simulink model "uav_plant_io"  (R2026a)
settings: Solver=ode4  StopTime=50  FixedStep=0.004
undefined symbols (not defined in the file or in its folder): controlParams, eQ, eT, GravityAcc, kQ, kT, Mass, minPWM, rotorsSpeedDown, rotorsSpeedUp, SampleTime, uavParam
libraries: slpidlib x24, simulink x11, robotcorelib x4, matrix_library x4, aerolibasang x4, aerolibobsolete x1, uavutilslib x1
(part 1 of 3)
settings Model: Creator=abutf  LastModifiedBy=Aaron

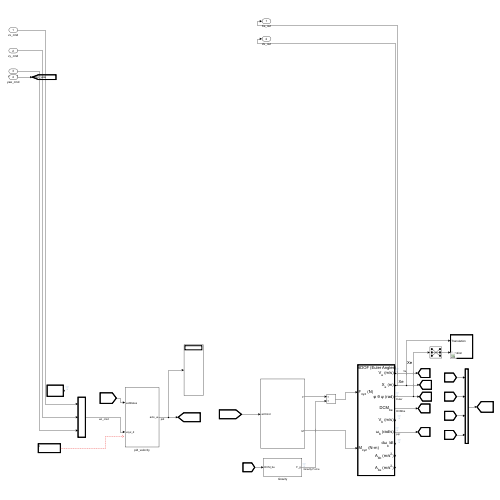
[thumbnail: Simulink's stored preview of the top-level diagram]
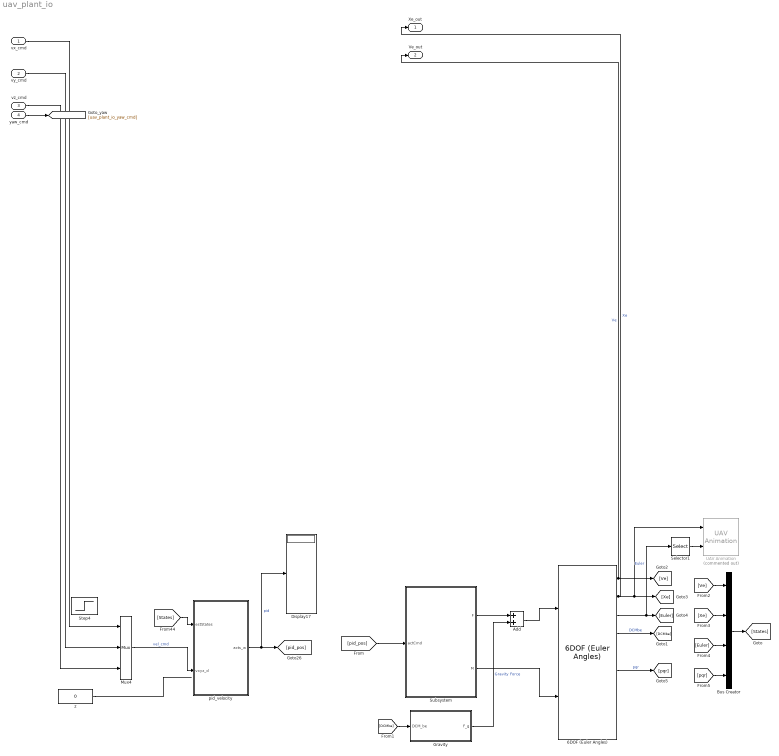
== system uav_plant_io ==
  vx_cmd : Inport
  vy_cmd : Inport  Port=2
  vz_cmd : Inport  Port=3
  yaw_cmd : Inport  Port=4
  6DOF (Euler Angles) : aerolibobsolete/6DOF (Euler Angles)  units=Metric (MKS)  mtype=Fixed  rep=Euler Angles  xme_0=[0, 0, 0]  Vm_0=[0 0 0]  eul_0=[0 0 0]  pm_0=[0 0 0]  mass_0=Mass  mass_e=0.5  mass_f=2.0  inertia=momentInertia  inertia_e=eye(3)  inertia_f=2*eye(3)  k_quat=1.0  vre_flag=on  abi_flag=on  aMode=0  xme_statename=''  Vm_statename=''  eul_statename=''  quat_statename=''  pm_statename=''  mass_statename=''
  Add : Sum
  Bus Creator : BusCreator  Inputs=4
  Display17 : Display
  Gravity : Subsystem
  Mux4 : Mux  Inputs=3
  Selector1 : Selector  InputPortWidth=3  IndexOptions=Index vector (dialog)  Indices=[3 2 1]  OutputSizes=1
  Step4 : Step  Time=5  SampleTime=0
  Subsystem : Subsystem
  UAV Animation : uavutilslib/UAV Animation  Commented=on  NumUAV=1  DynamicUAVConfig=off  UAVType=Multirotor  UAVSize=5  UAVColor=[1 0 0]  UAVTrajectoryAlpha=1  AlwaysShowAnimation=on  AxisLimits=[-Inf Inf;-Inf Inf;-Inf Inf]  TrajectoryBufferSize=100000  InertialZDirection=Down  RotationFormat=Euler ZYX  DrawMarkers=off  SampleTime=-1
  pid_velocity : Subsystem
  z : Constant  Value=0
  Xe_out : Outport
  Ve_out : Outport  Port=2
  wires:
  Mux4/1 -> pid_velocity/2(vxyz_d)  "vel_cmd"
  z/1 -> ?
  [States] -> pid_velocity/1(estStates)
  pid_velocity/1(acts_w) -> [pid_pos], Display17/1  "pid"
  [pid_pos] -> Subsystem/1(actCmd)
  Add/1 -> 6DOF (Euler Angles)/1
  Subsystem/1(F) -> Add/1
  Gravity/1(F_g) -> Add/2  "Gravity Force"
  Subsystem/2(M) -> 6DOF (Euler Angles)/2
  Bus Creator/1 -> [States]
  6DOF (Euler Angles)/4 -> [DCMbe]  "DCMbe"
  [DCMbe] -> Gravity/1(DCM_be)
  6DOF (Euler Angles)/1 -> [Ve], Ve_out/1  "Ve"
  [Ve] -> Bus Creator/1
  [Xe] -> Bus Creator/2
  6DOF (Euler Angles)/3 -> Selector1/1, [Euler]  "Euler"
  [Euler] -> Bus Creator/3
  6DOF (Euler Angles)/6 -> [pqr]  "pqr"
  [pqr] -> Bus Creator/4
  6DOF (Euler Angles)/2 -> UAV Animation/1, [Xe], Xe_out/1  "Xe"
  Selector1/1 -> UAV Animation/2
  vx_cmd/1 -> Mux4/1
  vy_cmd/1 -> Mux4/2
  vz_cmd/1 -> Mux4/3
  yaw_cmd/1 -> [uav_plant_io_yaw_cmd]

== system uav_plant_io/Gravity ==
  DCM_be : Inport
  Constant : Constant  Value=[0 0 GravityAcc]'
  Display4 : Display
  Gain : Gain  Gain=Mass
  Matrix Multiply : Product  Multiplication=Matrix(*)
  F_g : Outport
  wires:
  Matrix Multiply/1 -> Gain/1
  Constant/1 -> Matrix Multiply/2
  DCM_be/1 -> Matrix Multiply/1
  Gain/1 -> Display4/1, F_g/1

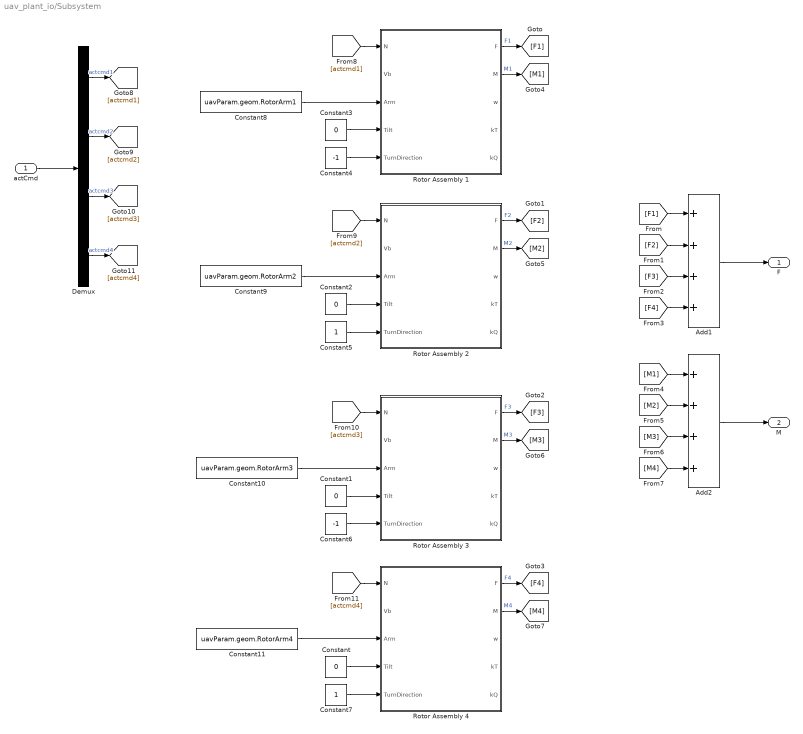
== system uav_plant_io/Subsystem ==
  actCmd : Inport
  Add1 : Sum  Inputs=++++
  Add2 : Sum  Inputs=++++
  Constant{,1..3} (4 alike) : Constant  Value=0
  Constant10 : Constant  Value=uavParam.geom.RotorArm3
  Constant11 : Constant  Value=uavParam.geom.RotorArm4
  Constant4 : Constant  Value=-1
  Constant5 : Constant
  Constant6 : Constant  Value=-1
  Constant7 : Constant
  Constant8 : Constant  Value=uavParam.geom.RotorArm1
  Constant9 : Constant  Value=uavParam.geom.RotorArm2
  Demux : Demux
  Rotor Assembly 1 : Subsystem
  Rotor Assembly 2 : Subsystem
  Rotor Assembly 3 : Subsystem
  Rotor Assembly 4 : Subsystem
  F : Outport
  M : Outport  Port=2
  wires:
  Constant10/1 -> Rotor Assembly 3/3(Arm)
  Add1/1 -> F/1
  ? -> Rotor Assembly 3/2(Vb)
  Constant6/1 -> Rotor Assembly 3/5(TurnDirection)
  Constant1/1 -> Rotor Assembly 3/4(Tilt)
  Add2/1 -> M/1
  Constant/1 -> Rotor Assembly 4/4(Tilt)
  Constant2/1 -> Rotor Assembly 2/4(Tilt)
  Constant3/1 -> Rotor Assembly 1/4(Tilt)
  Constant4/1 -> Rotor Assembly 1/5(TurnDirection)
  Constant5/1 -> Rotor Assembly 2/5(TurnDirection)
  Constant7/1 -> Rotor Assembly 4/5(TurnDirection)
  Constant8/1 -> Rotor Assembly 1/3(Arm)
  Constant9/1 -> Rotor Assembly 2/3(Arm)
  Constant11/1 -> Rotor Assembly 4/3(Arm)
  Rotor Assembly 1/1(F) -> [F1]  "F1"
  [F1] -> Add1/1
  Rotor Assembly 2/1(F) -> [F2]  "F2"
  [F2] -> Add1/2
  Rotor Assembly 3/1(F) -> [F3]  "F3"
  [F3] -> Add1/3
  Rotor Assembly 4/1(F) -> [F4]  "F4"
  [F4] -> Add1/4
  Rotor Assembly 1/2(M) -> [M1]  "M1"
  [M1] -> Add2/1
  Rotor Assembly 2/2(M) -> [M2]  "M2"
  [M2] -> Add2/2
  Rotor Assembly 3/2(M) -> [M3]  "M3"
  [M3] -> Add2/3
  Rotor Assembly 4/2(M) -> [M4]  "M4"
  [M4] -> Add2/4
  actCmd/1 -> Demux/1
  Demux/1 -> [actcmd1]  "actcmd1"
  [actcmd1] -> Rotor Assembly 1/1(N)
  Demux/2 -> [actcmd2]  "actcmd2"
  [actcmd2] -> Rotor Assembly 2/1(N)
  Demux/3 -> [actcmd3]  "actcmd3"
  [actcmd3] -> Rotor Assembly 3/1(N)
  Demux/4 -> [actcmd4]  "actcmd4"
  [actcmd4] -> Rotor Assembly 4/1(N)

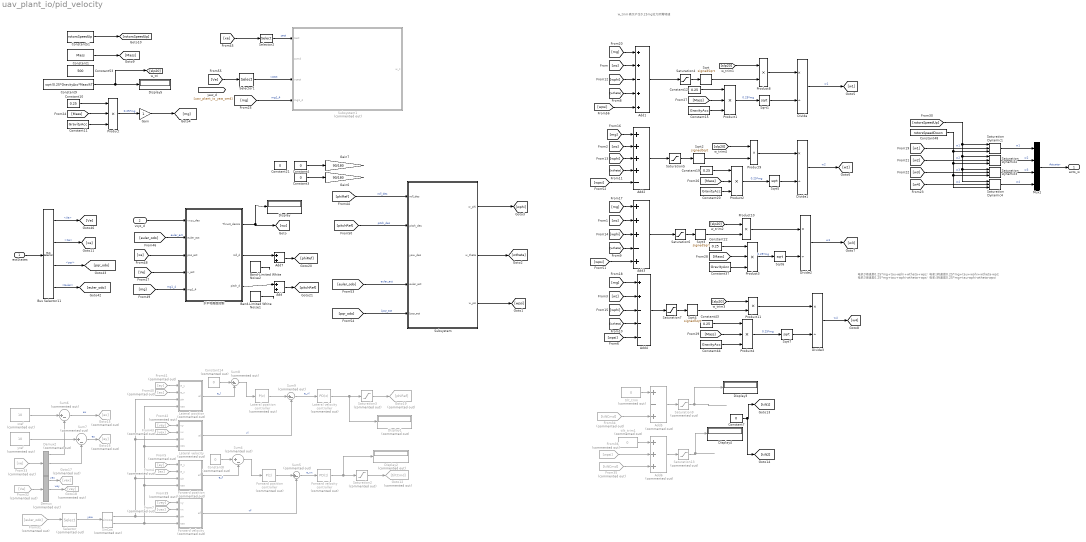
== system uav_plant_io/pid_velocity ==
  note: 电机1转速是0.25*mg+tau-wphi+wtheta+wpsi，
      | 电机2转速是0.25*mg+tau+wphi+wtheta-wpsi，
      | 电机3转速是0.25*mg+tau+wphi-wtheta+wpsi，
      | 电机4转速是0.25*mg+tau-wphi-wtheta-wpsi
  note: w_trim 表示产生0.25mg拉力所需转速
  estStates : Inport
  vxyz_d : Inport  Port=2
  Add : Sum
  Add1 : Sum  Inputs=++-++
  Add2 : Sum  Inputs=++++-
  Add3 : Sum  Inputs=+++-+
  Add4 : Sum  Inputs=++---
  Add5 : Sum  Commented=on  Inputs=+-+
  Add6 : Sum  Commented=on  Inputs=+++
  Add7 : Sum
  Band-Limited White Noise1 : simulink/Sources/Band-Limited White Noise  Cov=[0.000001]  Ts=SampleTime  seed=[23341]
  Band-Limited White Noise2 : simulink/Sources/Band-Limited White Noise  Cov=[0.000001]  Ts=SampleTime  seed=[2341]
  Bus Selector11 : BusSelector  OutputSignals=Ve,Xe,pqr,Euler
  Constant1 : Constant  Value=Mass  OutDataTypeStr=double
  Constant{10,12,19,22,43} (5 alike) : Constant  Value=0.25  OutDataTypeStr=double
  Constant{11,15,20,37,44} (5 alike) : Constant  Value=GravityAcc  OutDataTypeStr=double
  Constant14 : Constant  Commented=on  Value=0
  Constant{3..4,7,21} (4 alike) : Constant  Value=0  OutDataTypeStr=double
  Constant48 : Constant  Value=rotorsSpeedDown  OutDataTypeStr=double
  Constant51 : Constant  Value=rotorsSpeedUp  OutDataTypeStr=double
  Constant53 : Constant  Value=500
  Constant8 : Constant  Commented=on  Value=0
  Constant9 : Constant  Value=sqrt(0.25*GravityAcc*Mass/kT)
  Demux : Demux  Commented=on  Outputs=3
  Demux2 : Demux  Commented=on  Outputs=3
  Display{,3..5} (4 alike) : Display
  Display1 : Display  Commented=on
  Display2 : Display  Commented=on
  Divide{,1..3} (4 alike) : Product  Inputs=*/
  Forward position : Subsystem  Commented=on
  Forward position controller : slpidlib/PID Controller  Commented=on  Controller=P  Form=Parallel  TimeDomain=Discrete-time  UseExternalTs=off  SampleTime=-1  IntegratorMethod=Forward Euler  FilterMethod=Forward Euler  ControllerParametersSource=internal  P=1  I=controlParams.I_X  UseKiTs=off  D=0.741088334151374  UseExternalDerivativeSource=off  N=1.14081860742283  UseFilter=on  TunerSelectOption=Transfer Function Based (PID Tuner App)  InitialConditionSource=internal  InitialConditionForIntegrator=0  InitialConditionForFilter=0  DifferentiatorICPrevScaledInput=0  ExternalReset=none  TrackingMode=off  Kt=1  LimitOutput=off  SatLimitsSource=internal  UpperSaturationLimit=inf  LowerSaturationLimit=-inf  LinearizeAsGain=on  AntiWindupMode=none  Kb=1  LimitIntegrator=off  UpperIntegratorSaturationLimit=inf  LowerIntegratorSaturationLimit=-inf  POutMin=[]  POutMax=[]  IOutMin=[]  IOutMax=[]  DOutMin=[]  DOutMax=[]  NOutMin=[]  NOutMax=[]  SumOutMin=[]  SumOutMax=[]  SaturationOutMin=[]  SaturationOutMax=[]  PParamMin=[]  PParamMax=[]  IParamMin=[]  IParamMax=[]  DParamMin=[]  DParamMax=[]  NParamMin=[]  NParamMax=[]  KbParamMin=[]  KbParamMax=[]  KtParamMin=[]  KtParamMax=[]  KbOutMin=[]  KbOutMax=[]  KtOutMin=[]  KtOutMax=[]  IntegratorOutMin=[]  IntegratorOutMax=[]  FilterOutMin=[]  FilterOutMax=[]  SumI1OutMin=[]  SumI1OutMax=[]  SumI2OutMin=[]  SumI2OutMax=[]  SumI3OutMin=[]  SumI3OutMax=[]  SumI4OutMin=[]  SumI4OutMax=[]  SumDOutMin=[]  SumDOutMax=[]  DifferentiatorOutMin=[]  DifferentiatorOutMax=[]  FilterDiffOutCoefMin=[]  FilterDiffOutCoefMax=[]  ReciprocalOutMin=[]  ReciprocalOutMax=[]  SumDenOutMin=[]  SumDenOutMax=[]  SumNumOutMin=[]  SumNumOutMax=[]  DivideOutMin=[]  DivideOutMax=[]  UdiffTsProdOutMin=[]  UdiffTsProdOutMax=[]  NTsProdOutMin=[]  NTsProdOutMax=[]  UintegralTsProdOutMin=[]  UintegralTsProdOutMax=[]  UngainTsProdOutMin=[]  UngainTsProdOutMax=[]  ClampingZeroOutDataTypeStr=Inherit: Inherit via back propagation  ClampingZeroOutMin=[]  ClampingZeroOutMax=[]  FilterDenConstantOutDataTypeStr=Inherit: Inherit via back propagation  FilterDenConstantOutMin=[]  FilterDenConstantOutMax=[]  PCopyOutDataTypeStr=Inherit: Inherit via back propagation  PCopyOutMin=[]  PCopyOutMax=[]  NCopyOutDataTypeStr=Inherit: Inherit via back propagation  NCopyOutMin=[]  NCopyOutMax=[]  IntegratorContinuousStateAttributes=''  IntegratorStateMustResolveToSignalObject=off  IntegratorRTWStateStorageClass=Auto  FilterContinuousStateAttributes=''  FilterStateMustResolveToSignalObject=off  FilterRTWStateStorageClass=Auto  ParallelPVariant=InternalParameters  IdealPVariant=Disabled  IVariant=Disabled  DVariant=Disabled  IntegratorVariant=Disabled  SatVariant=Disabled  AWVariant=Disabled  PCopyVariant=Disabled  TRVariant=Disabled  FdbkBlocksVariant=Forward  IdealPFdbkVariant=Disabled  SatFdbkVariant=Disabled  DerivativeFilterVariant=Disabled  NVariant=Disabled  NCopyVariant=Disabled_SignalSpec  FilterICVariant=Disabled  IntegratorICVariant=Disabled  ExternalResetVariant=Disabled  TRSumVariant=Passthrough  SumFdbkVariant=Disabled  SumVariant=Passthrough_P  TsampFilterVariant=InternalTs  TsampNgainVariant=Passthrough  TsampIntegralVariant=Disabled_SignalSpec  ExternalSaturationOutDataTypeStr=Inherit: Same as second input  DerivativeSourceVariant=Disabled  PreIntVariant=InternalPreInt
  Forward velocity : Subsystem  Commented=on
  Forward velocity controller : slpidlib/PID Controller  Commented=on  Controller=PD  Form=Parallel  TimeDomain=Discrete-time  UseExternalTs=off  SampleTime=-1  IntegratorMethod=Forward Euler  FilterMethod=Forward Euler  ControllerParametersSource=internal  P=10  I=0  UseKiTs=off  D=0.1  UseExternalDerivativeSource=off  N=20  UseFilter=on  TunerSelectOption=Transfer Function Based (PID Tuner App)  InitialConditionSource=internal  InitialConditionForIntegrator=0  InitialConditionForFilter=0  DifferentiatorICPrevScaledInput=0  ExternalReset=none  TrackingMode=off  Kt=1  LimitOutput=off  SatLimitsSource=internal  UpperSaturationLimit=inf  LowerSaturationLimit=-inf  LinearizeAsGain=on  AntiWindupMode=none  Kb=1  LimitIntegrator=off  UpperIntegratorSaturationLimit=inf  LowerIntegratorSaturationLimit=-inf  POutMin=[]  POutMax=[]  IOutMin=[]  IOutMax=[]  DOutMin=[]  DOutMax=[]  NOutMin=[]  NOutMax=[]  SumOutMin=[]  SumOutMax=[]  SaturationOutMin=[]  SaturationOutMax=[]  PParamMin=[]  PParamMax=[]  IParamMin=[]  IParamMax=[]  DParamMin=[]  DParamMax=[]  NParamMin=[]  NParamMax=[]  KbParamMin=[]  KbParamMax=[]  KtParamMin=[]  KtParamMax=[]  KbOutMin=[]  KbOutMax=[]  KtOutMin=[]  KtOutMax=[]  IntegratorOutMin=[]  IntegratorOutMax=[]  FilterOutMin=[]  FilterOutMax=[]  SumI1OutMin=[]  SumI1OutMax=[]  SumI2OutMin=[]  SumI2OutMax=[]  SumI3OutMin=[]  SumI3OutMax=[]  SumI4OutMin=[]  SumI4OutMax=[]  SumDOutMin=[]  SumDOutMax=[]  DifferentiatorOutMin=[]  DifferentiatorOutMax=[]  FilterDiffOutCoefMin=[]  FilterDiffOutCoefMax=[]  ReciprocalOutMin=[]  ReciprocalOutMax=[]  SumDenOutMin=[]  SumDenOutMax=[]  SumNumOutMin=[]  SumNumOutMax=[]  DivideOutMin=[]  DivideOutMax=[]  UdiffTsProdOutMin=[]  UdiffTsProdOutMax=[]  NTsProdOutMin=[]  NTsProdOutMax=[]  UintegralTsProdOutMin=[]  UintegralTsProdOutMax=[]  UngainTsProdOutMin=[]  UngainTsProdOutMax=[]  ClampingZeroOutDataTypeStr=Inherit: Inherit via back propagation  ClampingZeroOutMin=[]  ClampingZeroOutMax=[]  FilterDenConstantOutDataTypeStr=Inherit: Inherit via back propagation  FilterDenConstantOutMin=[]  FilterDenConstantOutMax=[]  PCopyOutDataTypeStr=Inherit: Inherit via back propagation  PCopyOutMin=[]  PCopyOutMax=[]  NCopyOutDataTypeStr=Inherit: Inherit via back propagation  NCopyOutMin=[]  NCopyOutMax=[]  IntegratorContinuousStateAttributes=''  IntegratorStateMustResolveToSignalObject=off  IntegratorRTWStateStorageClass=Auto  FilterContinuousStateAttributes=''  FilterStateMustResolveToSignalObject=off  FilterRTWStateStorageClass=Auto  ParallelPVariant=InternalParameters  IdealPVariant=Disabled  IVariant=Disabled  DVariant=InternalParameters  IntegratorVariant=Disabled  SatVariant=Disabled  AWVariant=Disabled  PCopyVariant=Disabled  TRVariant=Disabled  FdbkBlocksVariant=Forward  IdealPFdbkVariant=Disabled  SatFdbkVariant=Disabled  DerivativeFilterVariant=ForwardEulerFilter  NVariant=InternalParameters  NCopyVariant=Disabled  FilterICVariant=InternalICsFilter  IntegratorICVariant=Disabled  ExternalResetVariant=Disabled  TRSumVariant=Passthrough  SumFdbkVariant=Disabled  SumVariant=Sum_PD  TsampFilterVariant=InternalTs  TsampNgainVariant=Passthrough  TsampIntegralVariant=Disabled_SignalSpec  ExternalSaturationOutDataTypeStr=Inherit: Same as second input  DerivativeSourceVariant=ErrorSignal  PreIntVariant=InternalPreInt
  From31 : From  Commented=on  GotoTag=euler_odo
  From32 : From  Commented=on  GotoTag=Ve
  From33 : From  Commented=on  GotoTag=xe
  From34 : From  Commented=on  GotoTag=tiltCmd
  From35 : From  Commented=on  GotoTag=tiltCmd
  From36 : From  Commented=on  GotoTag=wpsi
  From39 : From  Commented=on  GotoTag=vey
  From4 : From  Commented=on  GotoTag=ex
  From40 : From  Commented=on  GotoTag=ex
  From41 : From  Commented=on  GotoTag=ey
  From42 : From  Commented=on  GotoTag=vey
  From43 : From  Commented=on  GotoTag=vex
  From5 : From  Commented=on  GotoTag=ey
  From7 : From  Commented=on  GotoTag=vex
  Gain : Gain
  Gain6 : Gain  Gain=90/180
  Gain7 : Gain  Gain=90/180
  Goto12 : Goto  Commented=on  GotoTag=tiltCmd
  Goto15 : Goto  Commented=on  GotoTag=ex
  Goto16 : Goto  Commented=on  GotoTag=ey
  Goto17 : Goto  Commented=on  GotoTag=vex
  Goto18 : Goto  Commented=on  GotoTag=vey
  Goto19 : Goto  Commented=on  GotoTag=phiRef
  Lateral position : Subsystem  Commented=on
  Lateral position controller : slpidlib/PID Controller  Commented=on  Controller=P  Form=Parallel  TimeDomain=Discrete-time  UseExternalTs=off  SampleTime=-1  IntegratorMethod=Forward Euler  FilterMethod=Forward Euler  ControllerParametersSource=internal  P=1  I=controlParams.I_Y  UseKiTs=off  D=0.20966837124708  UseExternalDerivativeSource=off  N=1.18305565097938  UseFilter=on  TunerSelectOption=Transfer Function Based (PID Tuner App)  InitialConditionSource=internal  InitialConditionForIntegrator=0  InitialConditionForFilter=0  DifferentiatorICPrevScaledInput=0  ExternalReset=none  TrackingMode=off  Kt=1  LimitOutput=off  SatLimitsSource=internal  UpperSaturationLimit=0.4  LowerSaturationLimit=-0.4  LinearizeAsGain=on  AntiWindupMode=clamping  Kb=1  LimitIntegrator=off  UpperIntegratorSaturationLimit=inf  LowerIntegratorSaturationLimit=-inf  POutMin=[]  POutMax=[]  IOutMin=[]  IOutMax=[]  DOutMin=[]  DOutMax=[]  NOutMin=[]  NOutMax=[]  SumOutMin=[]  SumOutMax=[]  SaturationOutMin=[]  SaturationOutMax=[]  PParamMin=[]  PParamMax=[]  IParamMin=[]  IParamMax=[]  DParamMin=[]  DParamMax=[]  NParamMin=[]  NParamMax=[]  KbParamMin=[]  KbParamMax=[]  KtParamMin=[]  KtParamMax=[]  KbOutMin=[]  KbOutMax=[]  KtOutMin=[]  KtOutMax=[]  IntegratorOutMin=[]  IntegratorOutMax=[]  FilterOutMin=[]  FilterOutMax=[]  SumI1OutMin=[]  SumI1OutMax=[]  SumI2OutMin=[]  SumI2OutMax=[]  SumI3OutMin=[]  SumI3OutMax=[]  SumI4OutMin=[]  SumI4OutMax=[]  SumDOutMin=[]  SumDOutMax=[]  DifferentiatorOutMin=[]  DifferentiatorOutMax=[]  FilterDiffOutCoefMin=[]  FilterDiffOutCoefMax=[]  ReciprocalOutMin=[]  ReciprocalOutMax=[]  SumDenOutMin=[]  SumDenOutMax=[]  SumNumOutMin=[]  SumNumOutMax=[]  DivideOutMin=[]  DivideOutMax=[]  UdiffTsProdOutMin=[]  UdiffTsProdOutMax=[]  NTsProdOutMin=[]  NTsProdOutMax=[]  UintegralTsProdOutMin=[]  UintegralTsProdOutMax=[]  UngainTsProdOutMin=[]  UngainTsProdOutMax=[]  ClampingZeroOutDataTypeStr=Inherit: Inherit via back propagation  ClampingZeroOutMin=[]  ClampingZeroOutMax=[]  FilterDenConstantOutDataTypeStr=Inherit: Inherit via back propagation  FilterDenConstantOutMin=[]  FilterDenConstantOutMax=[]  PCopyOutDataTypeStr=Inherit: Inherit via back propagation  PCopyOutMin=[]  PCopyOutMax=[]  NCopyOutDataTypeStr=Inherit: Inherit via back propagation  NCopyOutMin=[]  NCopyOutMax=[]  IntegratorContinuousStateAttributes=''  IntegratorStateMustResolveToSignalObject=off  IntegratorRTWStateStorageClass=Auto  FilterContinuousStateAttributes=''  FilterStateMustResolveToSignalObject=off  FilterRTWStateStorageClass=Auto  ParallelPVariant=InternalParameters  IdealPVariant=Disabled  IVariant=Disabled  DVariant=Disabled  IntegratorVariant=Disabled  SatVariant=Disabled  AWVariant=Disabled  PCopyVariant=Disabled  TRVariant=Disabled  FdbkBlocksVariant=Forward  IdealPFdbkVariant=Disabled  SatFdbkVariant=Disabled  DerivativeFilterVariant=Disabled  NVariant=Disabled  NCopyVariant=Disabled_SignalSpec  FilterICVariant=Disabled  IntegratorICVariant=Disabled  ExternalResetVariant=Disabled  TRSumVariant=Passthrough  SumFdbkVariant=Disabled  SumVariant=Passthrough_P  TsampFilterVariant=InternalTs  TsampNgainVariant=Passthrough  TsampIntegralVariant=Disabled_SignalSpec  ExternalSaturationOutDataTypeStr=Inherit: Same as second input  DerivativeSourceVariant=Disabled  PreIntVariant=InternalPreInt
  Lateral velocity : Subsystem  Commented=on
  "Lateral velocity controller " : slpidlib/PID Controller  Commented=on  Controller=PD  Form=Parallel  TimeDomain=Discrete-time  UseExternalTs=off  SampleTime=-1  IntegratorMethod=Forward Euler  FilterMethod=Forward Euler  ControllerParametersSource=internal  P=10  I=0  UseKiTs=off  D=0.1  UseExternalDerivativeSource=off  N=20  UseFilter=on  TunerSelectOption=Transfer Function Based (PID Tuner App)  InitialConditionSource=internal  InitialConditionForIntegrator=0  InitialConditionForFilter=0  DifferentiatorICPrevScaledInput=0  ExternalReset=none  TrackingMode=off  Kt=1  LimitOutput=off  SatLimitsSource=internal  UpperSaturationLimit=inf  LowerSaturationLimit=-inf  LinearizeAsGain=on  AntiWindupMode=none  Kb=1  LimitIntegrator=off  UpperIntegratorSaturationLimit=inf  LowerIntegratorSaturationLimit=-inf  POutMin=[]  POutMax=[]  IOutMin=[]  IOutMax=[]  DOutMin=[]  DOutMax=[]  NOutMin=[]  NOutMax=[]  SumOutMin=[]  SumOutMax=[]  SaturationOutMin=[]  SaturationOutMax=[]  PParamMin=[]  PParamMax=[]  IParamMin=[]  IParamMax=[]  DParamMin=[]  DParamMax=[]  NParamMin=[]  NParamMax=[]  KbParamMin=[]  KbParamMax=[]  KtParamMin=[]  KtParamMax=[]  KbOutMin=[]  KbOutMax=[]  KtOutMin=[]  KtOutMax=[]  IntegratorOutMin=[]  IntegratorOutMax=[]  FilterOutMin=[]  FilterOutMax=[]  SumI1OutMin=[]  SumI1OutMax=[]  SumI2OutMin=[]  SumI2OutMax=[]  SumI3OutMin=[]  SumI3OutMax=[]  SumI4OutMin=[]  SumI4OutMax=[]  SumDOutMin=[]  SumDOutMax=[]  DifferentiatorOutMin=[]  DifferentiatorOutMax=[]  FilterDiffOutCoefMin=[]  FilterDiffOutCoefMax=[]  ReciprocalOutMin=[]  ReciprocalOutMax=[]  SumDenOutMin=[]  SumDenOutMax=[]  SumNumOutMin=[]  SumNumOutMax=[]  DivideOutMin=[]  DivideOutMax=[]  UdiffTsProdOutMin=[]  UdiffTsProdOutMax=[]  NTsProdOutMin=[]  NTsProdOutMax=[]  UintegralTsProdOutMin=[]  UintegralTsProdOutMax=[]  UngainTsProdOutMin=[]  UngainTsProdOutMax=[]  ClampingZeroOutDataTypeStr=Inherit: Inherit via back propagation  ClampingZeroOutMin=[]  ClampingZeroOutMax=[]  FilterDenConstantOutDataTypeStr=Inherit: Inherit via back propagation  FilterDenConstantOutMin=[]  FilterDenConstantOutMax=[]  PCopyOutDataTypeStr=Inherit: Inherit via back propagation  PCopyOutMin=[]  PCopyOutMax=[]  NCopyOutDataTypeStr=Inherit: Inherit via back propagation  NCopyOutMin=[]  NCopyOutMax=[]  IntegratorContinuousStateAttributes=''  IntegratorStateMustResolveToSignalObject=off  IntegratorRTWStateStorageClass=Auto  FilterContinuousStateAttributes=''  FilterStateMustResolveToSignalObject=off  FilterRTWStateStorageClass=Auto  ParallelPVariant=InternalParameters  IdealPVariant=Disabled  IVariant=Disabled  DVariant=InternalParameters  IntegratorVariant=Disabled  SatVariant=Disabled  AWVariant=Disabled  PCopyVariant=Disabled  TRVariant=Disabled  FdbkBlocksVariant=Forward  IdealPFdbkVariant=Disabled  SatFdbkVariant=Disabled  DerivativeFilterVariant=ForwardEulerFilter  NVariant=InternalParameters  NCopyVariant=Disabled  FilterICVariant=InternalICsFilter  IntegratorICVariant=Disabled  ExternalResetVariant=Disabled  TRSumVariant=Passthrough  SumFdbkVariant=Disabled  SumVariant=Sum_PD  TsampFilterVariant=InternalTs  TsampNgainVariant=Passthrough  TsampIntegralVariant=Disabled_SignalSpec  ExternalSaturationOutDataTypeStr=Inherit: Same as second input  DerivativeSourceVariant=ErrorSignal  PreIntVariant=InternalPreInt
  Mux1 : Mux
  Product{,1..4} (5 alike) : Product  Inputs=3
  Product{8..11} (4 alike) : Product
  Saturation Dynamic{1..4} (4 alike) : simulink/Discontinuities/Saturation Dynamic  OutMin=[]  OutMax=[]  OutDataTypeStr=double  OutDataType=fixdt(1, 16)  OutScaling=2^-10  DoSatur=off
  Saturation13 : Saturate  Commented=on  UpperLimit=0.3  LowerLimit=0
  Saturation2 : Saturate  Commented=on  UpperLimit=0.75  LowerLimit=-0.75
  Saturation3 : Saturate  Commented=on  UpperLimit=0.75  LowerLimit=-0.75
  Saturation{4..7} (4 alike) : Saturate  UpperLimit=inf  LowerLimit=0
  Saturation9 : Saturate  Commented=on  UpperLimit=0.3  LowerLimit=0
  Selector : Selector  Commented=on  InputPortWidth=3  IndexOptions=Index vector (dialog)  Indices=[3]  OutputSizes=1
  Selector1 : Selector  InputPortWidth=3  IndexOptions=Index vector (dialog)  Indices=[3]  OutputSizes=1
  Selector2 : Selector  InputPortWidth=3  IndexOptions=Index vector (dialog)  Indices=[3]  OutputSizes=1
  SinCos : Trigonometry  Commented=on  Operator=sincos
  Sqrt{,2..4} (4 alike) : Sqrt  Operator=signedSqrt
  Sqrt{1,5..7} (4 alike) : Sqrt
  Subsystem : Subsystem
  Subsystem1 : Subsystem  Commented=on
  Sum{4..9} (6 alike) : Sum  Commented=on  Inputs=|+-
  tilt_trim : Constant  Commented=on  Value=0
  tilt_trim1 : Constant  Commented=on  Value=0
  xref : Constant  Commented=on  Value=10  OutDataTypeStr=boolean
  yref : Constant  Commented=on  Value=10  OutDataTypeStr=boolean
  水平和高度控制 : Subsystem
  acts_w : Outport
  wires:
  Add7/1 -> [phiRef]
  Band-Limited White Noise2/1 -> ?
  Band-Limited White Noise1/1 -> ?
  Add/1 -> [pitchRef]
  Gain/1 -> [mg]
  Constant7/1 -> [tilt1], [tilt2]
  水平和高度控制/3(pitch_d) -> Add/1
  [mg] -> 水平和高度控制/5(mg1_4)  "mg1_4"
  [mg] -> Subsystem1/4(mg1_4)  "mg1_4"
  Selector1/1 -> Subsystem1/3(vzact)  "vzact"
  ? -> Subsystem1/2(zcmd)  "zcmd"
  Selector2/1 -> Subsystem1/1(zact)  "zact"
  水平和高度控制/1(Thrust_desire) -> [wz], Display/1
  vxyz_d/1 -> 水平和高度控制/1(vxyz_des)
  水平和高度控制/2(roll_d) -> Add7/1
  [xe] -> 水平和高度控制/3(pos_act)
  [Ve] -> 水平和高度控制/4(v_act)
  [euler_odo] -> 水平和高度控制/2(euler_act)  "euler_act"
  Subsystem/3(w_psi) -> [wpsi]
  Subsystem/2(w_theta) -> [wtheta]
  Subsystem/1(w_phi) -> [wphi]
  [pqr_odo] -> Subsystem/5("[pqr_act")  "[pqr_act"
  [euler_odo] -> Subsystem/4(euler_act)  "euler_act"
  [pitchRef] -> Subsystem/2(pitch_des)  "pitch_des"
  [phiRef] -> Subsystem/1(roll_des)  "roll_des"
  Bus Selector11/4 -> [euler_odo]  "<Euler>"
  Bus Selector11/3 -> [pqr_odo]  "<pqr>"
  Bus Selector11/2 -> [xe]  "<Xe>"
  Bus Selector11/1 -> [Ve]  "<Ve>"
  Constant51/1 -> [rotorsSpeedUp]
  Constant9/1 -> [slp20], Display5/1
  Constant1/1 -> [Mass]
  Mux1/1 -> acts_w/1  "Actuator"
  estStates/1 -> Bus Selector11/1
  [w2] -> Saturation Dynamic2/2  "w2"
  [w4] -> Saturation Dynamic4/2  "w4"
  [w3] -> Saturation Dynamic3/2  "w3"
  [w1] -> Saturation Dynamic1/2  "w1"
  [rotorsSpeedUp] -> Saturation Dynamic1/1, Saturation Dynamic2/1, Saturation Dynamic4/1, Saturation Dynamic3/1
  Constant48/1 -> Saturation Dynamic1/3, Saturation Dynamic2/3, Saturation Dynamic4/3, Saturation Dynamic3/3
  [slp20] -> Product11/1
  [slp20] -> Product10/1
  [slp20] -> Product9/1
  [slp20] -> Product8/1
  Sqrt7/1 -> Divide3/2
  Constant44/1 -> Product4/3
  [Mass] -> Product4/2
  Constant43/1 -> Product4/1
  Product4/1 -> Sqrt7/1  "0.25*mg"
  Product11/1 -> Divide3/1
  Product10/1 -> Divide2/1
  Product3/1 -> Sqrt6/1  "0.25*mg"
  Constant22/1 -> Product3/1
  [Mass] -> Product3/2
  Constant37/1 -> Product3/3
  Sqrt6/1 -> Divide2/2
  Sqrt5/1 -> Divide1/2
  Constant20/1 -> Product2/3
  [Mass] -> Product2/2
  Constant19/1 -> Product2/1
  Product2/1 -> Sqrt5/1  "0.25*mg"
  Product9/1 -> Divide1/1
  Product8/1 -> Divide/1
  Product1/1 -> Sqrt1/1  "0.25*mg"
  Constant12/1 -> Product1/1
  [Mass] -> Product1/2
  Constant15/1 -> Product1/3
  Sqrt1/1 -> Divide/2
  Constant11/1 -> Product/3
  [Mass] -> Product/2
  Constant10/1 -> Product/1
  Saturation Dynamic4/1 -> Mux1/4  "w4"
  Saturation Dynamic3/1 -> Mux1/3  "w3"
  Saturation Dynamic2/1 -> Mux1/2  "w2"
  Saturation Dynamic1/1 -> Mux1/1  "w1"
  [Ve] -> Selector1/1
  Divide3/1 -> [w4]  "w4"
  Divide2/1 -> [w3]  "w3"
  Divide1/1 -> [w2]  "w2"
  Divide/1 -> [w1]  "w1"
  [mg] -> Add4/1
  [mg] -> Add2/1
  [mg] -> Add3/1
  [mg] -> Add1/1
  Product/1 -> Gain/1  "0.25*mg"
  [wphi] -> Add4/3
  [wphi] -> Add3/3
  [wphi] -> Add2/3
  [wphi] -> Add1/3
  [wtheta] -> Add2/4
  [wtheta] -> Add4/4
  [wtheta] -> Add3/4
  [wtheta] -> Add1/4
  [wpsi] -> Add2/5
  [wpsi] -> Add4/5
  [wpsi] -> Add1/5
  [wpsi] -> Add3/5
  [wz] -> Add4/2
  [wz] -> Add2/2
  [wz] -> Add3/2
  [wz] -> Add1/2
  Saturation4/1 -> Sqrt/1
  Saturation6/1 -> Sqrt3/1
  Add3/1 -> Saturation6/1
  Add4/1 -> Saturation7/1
  Sqrt/1 -> Product8/2
  Saturation5/1 -> Sqrt2/1
  Add2/1 -> Saturation5/1
  Sqrt4/1 -> Product11/2
  Add1/1 -> Saturation4/1
  Saturation7/1 -> Sqrt4/1
  Sqrt3/1 -> Product10/2
  Sqrt2/1 -> Product9/2
  Constant4/1 -> Gain7/1
  Constant3/1 -> Gain6/1
  Forward position/1(ef) -> Sum4/2  "e_f"
  Sum5/1 -> Forward velocity controller/1  "e_vx"
  Forward velocity controller/1 -> Display2/1, Saturation2/1
  Constant8/1 -> Sum4/1
  Sum4/1 -> Forward position controller/1
  Forward velocity/1(ef) -> Sum5/2  "vf"
  Forward position controller/1 -> Sum5/1
  Selector/1 -> SinCos/1  "yaw"
  SinCos/2 -> Lateral velocity/4(cos), Lateral position/4(cos), Forward position/4(cos), Forward velocity/4(cos)
  SinCos/1 -> Forward velocity/3(sin), Lateral position/3(sin), Lateral velocity/3(sin), Forward position/3(sin)
  From31/1 -> Selector/1
  From32/1 -> Demux/1
  From33/1 -> Demux2/1
  Demux2/1 -> Sum6/2
  Demux2/2 -> Sum7/2
  xref/1 -> Sum6/1
  yref/1 -> Sum7/1
  Saturation2/1 -> Goto12/1
  Saturation9/1 -> Display3/1
  From36/1 -> Add6/2
  tilt_trim1/1 -> Add6/1
  Saturation13/1 -> Display4/1
  From35/1 -> Add6/3
  tilt_trim/1 -> Add5/1
  ? -> Add5/2
  From34/1 -> Add5/3
  Add5/1 -> Saturation9/1
  Add6/1 -> Saturation13/1
  Sum8/1 -> Lateral position controller/1
  Lateral position/1(el) -> Sum8/2  "e_l"
  Constant14/1 -> Sum8/1
  Sum9/1 -> "Lateral velocity controller "/1  "e_vl"
  Lateral position controller/1 -> Sum9/1
  Lateral velocity/1(el) -> Sum9/2  "vl"
  Sum6/1 -> Goto15/1  "ex"
  From4/1 -> Forward position/2(e_x)
  Sum7/1 -> Goto16/1  "ey"
  From5/1 -> Forward position/1(e_y)
  Demux/1 -> Goto17/1  "vex"
  From7/1 -> Forward velocity/2(vx)
  Demux/2 -> Goto18/1  "vey"
  From39/1 -> Forward velocity/1(vy)
  From40/1 -> Lateral position/2(e_x)
  From41/1 -> Lateral position/1(e_y)
  From42/1 -> Lateral velocity/1(vy)
  From43/1 -> Lateral velocity/2(vx)
  "Lateral velocity controller "/1 -> Saturation3/1, Display1/1
  [xe] -> Selector2/1
  Saturation3/1 -> Goto19/1

== system uav_plant_io/Subsystem/Rotor Assembly 1 ==
  note: RotorArm1=[ 0.375 0.375 0];
  N : Inport
  Vb : Inport  Port=2
  Arm : Inport  Port=3
  Tilt : Inport  Port=4
  TurnDirection : Inport  Port=5
  Adjust Force/Moment to Body Frame : Subsystem
  Display{2,7,9..12} (6 alike) : Display
  Gain : Gain  Commented=on  Gain=2*pi
  Gain1 : Gain  Commented=on  Gain=uavParam.motor.RPMMAX/60
  "Incidence, Sideslip, & Airspeed" : aerolibasang/Incidence, Sideslip, & Airspeed
  Saturation : Saturate  Commented=on  UpperLimit=1  LowerLimit=minPWM
  Saturation2 : Saturate  UpperLimit=rotorsSpeedUp  LowerLimit=rotorsSpeedDown
  Subsystem : Subsystem
  F : Outport
  M : Outport  Port=2
  w : Outport  Port=3
  kT : Outport  Port=4
  kQ : Outport  Port=5
  wires:
  Subsystem/4(kQ) -> Display11/1, kQ/1
  Subsystem/3(kT) -> Display10/1, kT/1
  "Incidence, Sideslip, & Airspeed"/3 -> Subsystem/1(Va), Display12/1  "airspeed"
  Subsystem/2(Mxyz) -> Display7/1, Adjust Force/Moment to Body Frame/2(Mmotor)
  Adjust Force/Moment to Body Frame/2(Mbody) -> M/1
  Arm/1 -> Adjust Force/Moment to Body Frame/5(Arm1)
  Saturation2/1 -> Subsystem/2(Omega), Display2/1, w/1
  N/1 -> Saturation2/1
  Subsystem/1(Fxyz) -> Display9/1, Adjust Force/Moment to Body Frame/1(Fmotor)
  Tilt/1 -> Adjust Force/Moment to Body Frame/3(Tilt)
  Gain1/1 -> Gain/1  "W"
  Saturation/1 -> Gain1/1
  Vb/1 -> "Incidence, Sideslip, & Airspeed"/1
  Adjust Force/Moment to Body Frame/1(Fbody) -> F/1
  TurnDirection/1 -> Adjust Force/Moment to Body Frame/4(TurnDirection)

== system uav_plant_io/Subsystem/Rotor Assembly 2 ==
  note: RotorArm1=[ 0.375 0.375 0];
  N : Inport
  Vb : Inport  Port=2
  Arm : Inport  Port=3
  Tilt : Inport  Port=4
  TurnDirection : Inport  Port=5
  Adjust Force/Moment to Body Frame : Subsystem
  Display{2,7,9..12} (6 alike) : Display
  Gain : Gain  Commented=on  Gain=2*pi
  Gain1 : Gain  Commented=on  Gain=uavParam.motor.RPMMAX/60
  "Incidence, Sideslip, & Airspeed" : aerolibasang/Incidence, Sideslip, & Airspeed
  Saturation : Saturate  Commented=on  UpperLimit=1  LowerLimit=minPWM
  Saturation2 : Saturate  UpperLimit=rotorsSpeedUp  LowerLimit=rotorsSpeedDown
  Subsystem : Subsystem
  F : Outport
  M : Outport  Port=2
  w : Outport  Port=3
  kT : Outport  Port=4
  kQ : Outport  Port=5
  wires:
  TurnDirection/1 -> Adjust Force/Moment to Body Frame/4(TurnDirection)
  Adjust Force/Moment to Body Frame/1(Fbody) -> F/1
  Vb/1 -> "Incidence, Sideslip, & Airspeed"/1
  Saturation/1 -> Gain1/1
  Gain1/1 -> Gain/1  "W"
  Tilt/1 -> Adjust Force/Moment to Body Frame/3(Tilt)
  Subsystem/1(Fxyz) -> Adjust Force/Moment to Body Frame/1(Fmotor), Display9/1
  N/1 -> Saturation2/1
  Saturation2/1 -> w/1, Display2/1, Subsystem/2(Omega)
  Arm/1 -> Adjust Force/Moment to Body Frame/5(Arm1)
  Adjust Force/Moment to Body Frame/2(Mbody) -> M/1
  Subsystem/2(Mxyz) -> Adjust Force/Moment to Body Frame/2(Mmotor), Display7/1
  "Incidence, Sideslip, & Airspeed"/3 -> Display12/1, Subsystem/1(Va)  "airspeed"
  Subsystem/3(kT) -> kT/1, Display10/1
  Subsystem/4(kQ) -> kQ/1, Display11/1

== system uav_plant_io/Subsystem/Rotor Assembly 3 ==
  note: RotorArm1=[ 0.375 0.375 0];
  N : Inport
  Vb : Inport  Port=2
  Arm : Inport  Port=3
  Tilt : Inport  Port=4
  TurnDirection : Inport  Port=5
  Adjust Force/Moment to Body Frame : Subsystem
  Display{2,7,9..12} (6 alike) : Display
  Gain : Gain  Commented=on  Gain=2*pi
  Gain1 : Gain  Commented=on  Gain=uavParam.motor.RPMMAX/60
  "Incidence, Sideslip, & Airspeed" : aerolibasang/Incidence, Sideslip, & Airspeed
  Saturation : Saturate  Commented=on  UpperLimit=1  LowerLimit=minPWM
  Saturation2 : Saturate  UpperLimit=rotorsSpeedUp  LowerLimit=rotorsSpeedDown
  Subsystem : Subsystem
  F : Outport
  M : Outport  Port=2
  w : Outport  Port=3
  kT : Outport  Port=4
  kQ : Outport  Port=5
  wires:
  TurnDirection/1 -> Adjust Force/Moment to Body Frame/4(TurnDirection)
  Adjust Force/Moment to Body Frame/1(Fbody) -> F/1
  Vb/1 -> "Incidence, Sideslip, & Airspeed"/1
  Saturation/1 -> Gain1/1
  Gain1/1 -> Gain/1  "W"
  Tilt/1 -> Adjust Force/Moment to Body Frame/3(Tilt)
  Subsystem/1(Fxyz) -> Adjust Force/Moment to Body Frame/1(Fmotor), Display9/1
  N/1 -> Saturation2/1
  Saturation2/1 -> w/1, Display2/1, Subsystem/2(Omega)
  Arm/1 -> Adjust Force/Moment to Body Frame/5(Arm1)
  Adjust Force/Moment to Body Frame/2(Mbody) -> M/1
  Subsystem/2(Mxyz) -> Adjust Force/Moment to Body Frame/2(Mmotor), Display7/1
  "Incidence, Sideslip, & Airspeed"/3 -> Display12/1, Subsystem/1(Va)  "airspeed"
  Subsystem/3(kT) -> kT/1, Display10/1
  Subsystem/4(kQ) -> kQ/1, Display11/1

== system uav_plant_io/Subsystem/Rotor Assembly 4 ==
  note: RotorArm1=[ 0.375 0.375 0];
  N : Inport
  Vb : Inport  Port=2
  Arm : Inport  Port=3
  Tilt : Inport  Port=4
  TurnDirection : Inport  Port=5
  Adjust Force/Moment to Body Frame : Subsystem
  Display{2,7,9..12} (6 alike) : Display
  Gain : Gain  Commented=on  Gain=2*pi
  Gain1 : Gain  Commented=on  Gain=uavParam.motor.RPMMAX/60
  "Incidence, Sideslip, & Airspeed" : aerolibasang/Incidence, Sideslip, & Airspeed
  Saturation : Saturate  Commented=on  UpperLimit=1  LowerLimit=minPWM
  Saturation2 : Saturate  UpperLimit=rotorsSpeedUp  LowerLimit=rotorsSpeedDown
  Subsystem : Subsystem
  F : Outport
  M : Outport  Port=2
  w : Outport  Port=3
  kT : Outport  Port=4
  kQ : Outport  Port=5
  wires:
  Subsystem/4(kQ) -> Display11/1, kQ/1
  Subsystem/3(kT) -> Display10/1, kT/1
  "Incidence, Sideslip, & Airspeed"/3 -> Subsystem/1(Va), Display12/1  "airspeed"
  Subsystem/2(Mxyz) -> Display7/1, Adjust Force/Moment to Body Frame/2(Mmotor)
  Adjust Force/Moment to Body Frame/2(Mbody) -> M/1
  Arm/1 -> Adjust Force/Moment to Body Frame/5(Arm1)
  Saturation2/1 -> Subsystem/2(Omega), Display2/1, w/1
  N/1 -> Saturation2/1
  Subsystem/1(Fxyz) -> Display9/1, Adjust Force/Moment to Body Frame/1(Fmotor)
  Tilt/1 -> Adjust Force/Moment to Body Frame/3(Tilt)
  Gain1/1 -> Gain/1  "W"
  Saturation/1 -> Gain1/1
  Vb/1 -> "Incidence, Sideslip, & Airspeed"/1
  Adjust Force/Moment to Body Frame/1(Fbody) -> F/1
  TurnDirection/1 -> Adjust Force/Moment to Body Frame/4(TurnDirection)

== system uav_plant_io/pid_velocity/Forward position ==
  e_y : Inport
  e_x : Inport  Port=2
  sin : Inport  Port=3
  cos : Inport  Port=4
  Add : Sum
  Product : Product
  Product1 : Product
  ef : Outport
  wires:
  Add/1 -> ef/1
  Product1/1 -> Add/2
  Product/1 -> Add/1
  e_x/1 -> Product/2
  e_y/1 -> Product1/1
  sin/1 -> Product1/2
  cos/1 -> Product/1

== system uav_plant_io/pid_velocity/Forward velocity ==
  vy : Inport
  vx : Inport  Port=2
  sin : Inport  Port=3
  cos : Inport  Port=4
  Add : Sum
  Product : Product
  Product1 : Product
  ef : Outport
  wires:
  cos/1 -> Product/1
  sin/1 -> Product1/2
  vy/1 -> Product1/1
  vx/1 -> Product/2
  Product/1 -> Add/1
  Product1/1 -> Add/2
  Add/1 -> ef/1

== system uav_plant_io/pid_velocity/Lateral position ==
  e_y : Inport
  e_x : Inport  Port=2
  sin : Inport  Port=3
  cos : Inport  Port=4
  Add : Sum
  Gain : Gain  Gain=-1
  Product : Product
  Product1 : Product
  el : Outport
  wires:
  e_y/1 -> Product1/1
  e_x/1 -> Product/2
  sin/1 -> Product/1
  cos/1 -> Product1/2
  Product/1 -> Gain/1
  Product1/1 -> Add/2
  Add/1 -> el/1
  Gain/1 -> Add/1

== system uav_plant_io/pid_velocity/Lateral velocity ==
  vy : Inport
  vx : Inport  Port=2
  sin : Inport  Port=3
  cos : Inport  Port=4
  Add : Sum
  Gain : Gain  Gain=-1
  Product : Product
  Product1 : Product
  el : Outport
  wires:
  Gain/1 -> Add/1
  Add/1 -> el/1
  Product1/1 -> Add/2
  Product/1 -> Gain/1
  cos/1 -> Product1/2
  sin/1 -> Product/1
  vx/1 -> Product/2
  vy/1 -> Product1/1

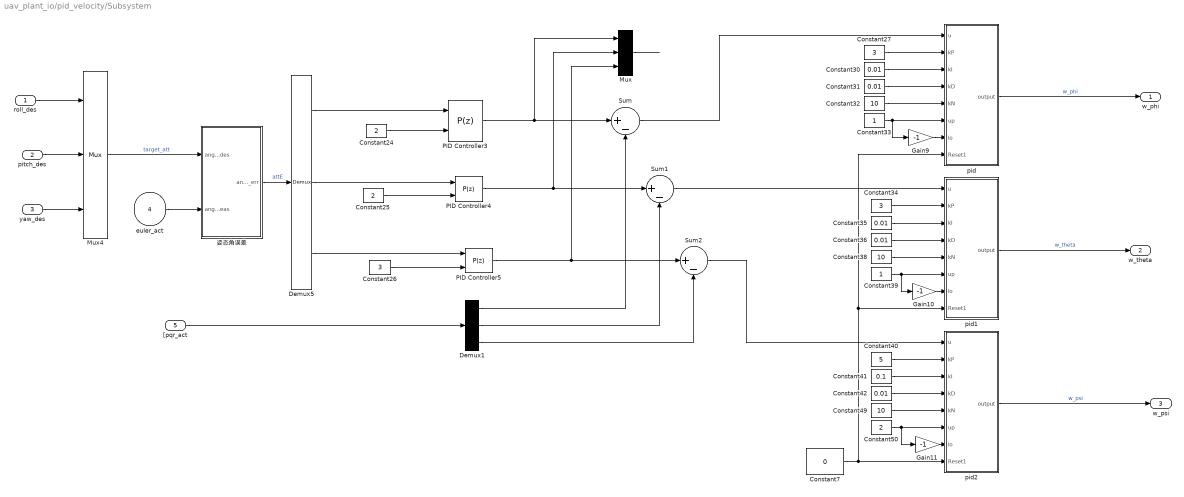
== system uav_plant_io/pid_velocity/Subsystem ==
  roll_des : Inport
  pitch_des : Inport  Port=2
  yaw_des : Inport  Port=3
  euler_act : Inport  Port=4
  "[pqr_act" : Inport  Port=5
  Constant24 : Constant  Value=2
  Constant25 : Constant  Value=2
  Constant26 : Constant  Value=3
  Constant27 : Constant  Value=3
  Constant{30..31,35..36,42} (5 alike) : Constant  Value=0.01
  Constant32 : Constant  Value=10
  Constant33 : Constant
  Constant34 : Constant  Value=3
  Constant38 : Constant  Value=10
  Constant39 : Constant
  Constant40 : Constant  Value=5
  Constant41 : Constant  Value=0.1
  Constant49 : Constant  Value=10
  Constant50 : Constant  Value=2
  Constant7 : Constant  Value=0  OutDataTypeStr=boolean
  Demux1 : Demux  Outputs=3
  Demux5 : Demux  Outputs=3
  Gain10 : Gain  Gain=-1
  Gain11 : Gain  Gain=-1
  Gain9 : Gain  Gain=-1
  Mux : Mux  Inputs=3
  Mux4 : Mux  Inputs=3
  PID Controller3 : slpidlib/PID Controller  Controller=P  Form=Parallel  TimeDomain=Discrete-time  UseExternalTs=off  SampleTime=-1  IntegratorMethod=Forward Euler  FilterMethod=Forward Euler  ControllerParametersSource=external  P=6  I=1  UseKiTs=off  D=0.2  UseExternalDerivativeSource=off  N=100  UseFilter=on  TunerSelectOption=Transfer Function Based (PID Tuner App)  InitialConditionSource=internal  InitialConditionForIntegrator=0  InitialConditionForFilter=0  DifferentiatorICPrevScaledInput=0  ExternalReset=none  TrackingMode=off  Kt=1  LimitOutput=off  SatLimitsSource=internal  UpperSaturationLimit=inf  LowerSaturationLimit=-inf  LinearizeAsGain=on  AntiWindupMode=none  Kb=1  LimitIntegrator=off  UpperIntegratorSaturationLimit=inf  LowerIntegratorSaturationLimit=-inf  POutMin=[]  POutMax=[]  IOutMin=[]  IOutMax=[]  DOutMin=[]  DOutMax=[]  NOutMin=[]  NOutMax=[]  SumOutMin=[]  SumOutMax=[]  SaturationOutMin=[]  SaturationOutMax=[]  PParamMin=[]  PParamMax=[]  IParamMin=[]  IParamMax=[]  DParamMin=[]  DParamMax=[]  NParamMin=[]  NParamMax=[]  KbParamMin=[]  KbParamMax=[]  KtParamMin=[]  KtParamMax=[]  KbOutMin=[]  KbOutMax=[]  KtOutMin=[]  KtOutMax=[]  IntegratorOutMin=[]  IntegratorOutMax=[]  FilterOutMin=[]  FilterOutMax=[]  SumI1OutMin=[]  SumI1OutMax=[]  SumI2OutMin=[]  SumI2OutMax=[]  SumI3OutMin=[]  SumI3OutMax=[]  SumI4OutMin=[]  SumI4OutMax=[]  SumDOutMin=[]  SumDOutMax=[]  DifferentiatorOutMin=[]  DifferentiatorOutMax=[]  FilterDiffOutCoefMin=[]  FilterDiffOutCoefMax=[]  ReciprocalOutMin=[]  ReciprocalOutMax=[]  SumDenOutMin=[]  SumDenOutMax=[]  SumNumOutMin=[]  SumNumOutMax=[]  DivideOutMin=[]  DivideOutMax=[]  UdiffTsProdOutMin=[]  UdiffTsProdOutMax=[]  NTsProdOutMin=[]  NTsProdOutMax=[]  UintegralTsProdOutMin=[]  UintegralTsProdOutMax=[]  UngainTsProdOutMin=[]  UngainTsProdOutMax=[]  ClampingZeroOutDataTypeStr=Inherit: Inherit via back propagation  ClampingZeroOutMin=[]  ClampingZeroOutMax=[]  FilterDenConstantOutDataTypeStr=Inherit: Inherit via back propagation  FilterDenConstantOutMin=[]  FilterDenConstantOutMax=[]  PCopyOutDataTypeStr=Inherit: Inherit via back propagation  PCopyOutMin=[]  PCopyOutMax=[]  NCopyOutDataTypeStr=Inherit: Inherit via back propagation  NCopyOutMin=[]  NCopyOutMax=[]  IntegratorContinuousStateAttributes=''  IntegratorStateMustResolveToSignalObject=off  IntegratorRTWStateStorageClass=Auto  FilterContinuousStateAttributes=''  FilterStateMustResolveToSignalObject=off  FilterRTWStateStorageClass=Auto  ParallelPVariant=ExternalParameters  IdealPVariant=Disabled  IVariant=Disabled  DVariant=Disabled  IntegratorVariant=Disabled  SatVariant=Disabled  AWVariant=Disabled  PCopyVariant=Disabled  TRVariant=Disabled  FdbkBlocksVariant=Forward  IdealPFdbkVariant=Disabled  SatFdbkVariant=Disabled  DerivativeFilterVariant=Disabled  NVariant=Disabled  NCopyVariant=Disabled_SignalSpec  FilterICVariant=Disabled  IntegratorICVariant=Disabled  ExternalResetVariant=Disabled  TRSumVariant=Passthrough  SumFdbkVariant=Disabled  SumVariant=Passthrough_P  TsampFilterVariant=InternalTs  TsampNgainVariant=Passthrough  TsampIntegralVariant=Disabled_SignalSpec  ExternalSaturationOutDataTypeStr=Inherit: Same as second input  DerivativeSourceVariant=Disabled  PreIntVariant=InternalPreInt
  PID Controller4 : slpidlib/PID Controller  Controller=P  Form=Parallel  TimeDomain=Discrete-time  UseExternalTs=off  SampleTime=-1  IntegratorMethod=Forward Euler  FilterMethod=Forward Euler  ControllerParametersSource=external  P=5  I=1  UseKiTs=off  D=0.2  UseExternalDerivativeSource=off  N=100  UseFilter=on  TunerSelectOption=Transfer Function Based (PID Tuner App)  InitialConditionSource=internal  InitialConditionForIntegrator=0  InitialConditionForFilter=0  DifferentiatorICPrevScaledInput=0  ExternalReset=none  TrackingMode=off  Kt=1  LimitOutput=off  SatLimitsSource=internal  UpperSaturationLimit=inf  LowerSaturationLimit=-inf  LinearizeAsGain=on  AntiWindupMode=none  Kb=1  LimitIntegrator=off  UpperIntegratorSaturationLimit=inf  LowerIntegratorSaturationLimit=-inf  POutMin=[]  POutMax=[]  IOutMin=[]  IOutMax=[]  DOutMin=[]  DOutMax=[]  NOutMin=[]  NOutMax=[]  SumOutMin=[]  SumOutMax=[]  SaturationOutMin=[]  SaturationOutMax=[]  PParamMin=[]  PParamMax=[]  IParamMin=[]  IParamMax=[]  DParamMin=[]  DParamMax=[]  NParamMin=[]  NParamMax=[]  KbParamMin=[]  KbParamMax=[]  KtParamMin=[]  KtParamMax=[]  KbOutMin=[]  KbOutMax=[]  KtOutMin=[]  KtOutMax=[]  IntegratorOutMin=[]  IntegratorOutMax=[]  FilterOutMin=[]  FilterOutMax=[]  SumI1OutMin=[]  SumI1OutMax=[]  SumI2OutMin=[]  SumI2OutMax=[]  SumI3OutMin=[]  SumI3OutMax=[]  SumI4OutMin=[]  SumI4OutMax=[]  SumDOutMin=[]  SumDOutMax=[]  DifferentiatorOutMin=[]  DifferentiatorOutMax=[]  FilterDiffOutCoefMin=[]  FilterDiffOutCoefMax=[]  ReciprocalOutMin=[]  ReciprocalOutMax=[]  SumDenOutMin=[]  SumDenOutMax=[]  SumNumOutMin=[]  SumNumOutMax=[]  DivideOutMin=[]  DivideOutMax=[]  UdiffTsProdOutMin=[]  UdiffTsProdOutMax=[]  NTsProdOutMin=[]  NTsProdOutMax=[]  UintegralTsProdOutMin=[]  UintegralTsProdOutMax=[]  UngainTsProdOutMin=[]  UngainTsProdOutMax=[]  ClampingZeroOutDataTypeStr=Inherit: Inherit via back propagation  ClampingZeroOutMin=[]  ClampingZeroOutMax=[]  FilterDenConstantOutDataTypeStr=Inherit: Inherit via back propagation  FilterDenConstantOutMin=[]  FilterDenConstantOutMax=[]  PCopyOutDataTypeStr=Inherit: Inherit via back propagation  PCopyOutMin=[]  PCopyOutMax=[]  NCopyOutDataTypeStr=Inherit: Inherit via back propagation  NCopyOutMin=[]  NCopyOutMax=[]  IntegratorContinuousStateAttributes=''  IntegratorStateMustResolveToSignalObject=off  IntegratorRTWStateStorageClass=Auto  FilterContinuousStateAttributes=''  FilterStateMustResolveToSignalObject=off  FilterRTWStateStorageClass=Auto  ParallelPVariant=ExternalParameters  IdealPVariant=Disabled  IVariant=Disabled  DVariant=Disabled  IntegratorVariant=Disabled  SatVariant=Disabled  AWVariant=Disabled  PCopyVariant=Disabled  TRVariant=Disabled  FdbkBlocksVariant=Forward  IdealPFdbkVariant=Disabled  SatFdbkVariant=Disabled  DerivativeFilterVariant=Disabled  NVariant=Disabled  NCopyVariant=Disabled_SignalSpec  FilterICVariant=Disabled  IntegratorICVariant=Disabled  ExternalResetVariant=Disabled  TRSumVariant=Passthrough  SumFdbkVariant=Disabled  SumVariant=Passthrough_P  TsampFilterVariant=InternalTs  TsampNgainVariant=Passthrough  TsampIntegralVariant=Disabled_SignalSpec  ExternalSaturationOutDataTypeStr=Inherit: Same as second input  DerivativeSourceVariant=Disabled  PreIntVariant=InternalPreInt
  PID Controller5 : slpidlib/PID Controller  Controller=P  Form=Parallel  TimeDomain=Discrete-time  UseExternalTs=off  SampleTime=-1  IntegratorMethod=Forward Euler  FilterMethod=Forward Euler  ControllerParametersSource=external  P=3  I=0.0593544486366272  UseKiTs=off  D=12.4048497936965  UseExternalDerivativeSource=off  N=6.75214061700394  UseFilter=on  TunerSelectOption=Transfer Function Based (PID Tuner App)  InitialConditionSource=internal  InitialConditionForIntegrator=0  InitialConditionForFilter=0  DifferentiatorICPrevScaledInput=0  ExternalReset=none  TrackingMode=off  Kt=1  LimitOutput=off  SatLimitsSource=internal  UpperSaturationLimit=inf  LowerSaturationLimit=-inf  LinearizeAsGain=on  AntiWindupMode=none  Kb=1  LimitIntegrator=off  UpperIntegratorSaturationLimit=inf  LowerIntegratorSaturationLimit=-inf  POutMin=[]  POutMax=[]  IOutMin=[]  IOutMax=[]  DOutMin=[]  DOutMax=[]  NOutMin=[]  NOutMax=[]  SumOutMin=[]  SumOutMax=[]  SaturationOutMin=[]  SaturationOutMax=[]  PParamMin=[]  PParamMax=[]  IParamMin=[]  IParamMax=[]  DParamMin=[]  DParamMax=[]  NParamMin=[]  NParamMax=[]  KbParamMin=[]  KbParamMax=[]  KtParamMin=[]  KtParamMax=[]  KbOutMin=[]  KbOutMax=[]  KtOutMin=[]  KtOutMax=[]  IntegratorOutMin=[]  IntegratorOutMax=[]  FilterOutMin=[]  FilterOutMax=[]  SumI1OutMin=[]  SumI1OutMax=[]  SumI2OutMin=[]  SumI2OutMax=[]  SumI3OutMin=[]  SumI3OutMax=[]  SumI4OutMin=[]  SumI4OutMax=[]  SumDOutMin=[]  SumDOutMax=[]  DifferentiatorOutMin=[]  DifferentiatorOutMax=[]  FilterDiffOutCoefMin=[]  FilterDiffOutCoefMax=[]  ReciprocalOutMin=[]  ReciprocalOutMax=[]  SumDenOutMin=[]  SumDenOutMax=[]  SumNumOutMin=[]  SumNumOutMax=[]  DivideOutMin=[]  DivideOutMax=[]  UdiffTsProdOutMin=[]  UdiffTsProdOutMax=[]  NTsProdOutMin=[]  NTsProdOutMax=[]  UintegralTsProdOutMin=[]  UintegralTsProdOutMax=[]  UngainTsProdOutMin=[]  UngainTsProdOutMax=[]  ClampingZeroOutDataTypeStr=Inherit: Inherit via back propagation  ClampingZeroOutMin=[]  ClampingZeroOutMax=[]  FilterDenConstantOutDataTypeStr=Inherit: Inherit via back propagation  FilterDenConstantOutMin=[]  FilterDenConstantOutMax=[]  PCopyOutDataTypeStr=Inherit: Inherit via back propagation  PCopyOutMin=[]  PCopyOutMax=[]  NCopyOutDataTypeStr=Inherit: Inherit via back propagation  NCopyOutMin=[]  NCopyOutMax=[]  IntegratorContinuousStateAttributes=''  IntegratorStateMustResolveToSignalObject=off  IntegratorRTWStateStorageClass=Auto  FilterContinuousStateAttributes=''  FilterStateMustResolveToSignalObject=off  FilterRTWStateStorageClass=Auto  ParallelPVariant=ExternalParameters  IdealPVariant=Disabled  IVariant=Disabled  DVariant=Disabled  IntegratorVariant=Disabled  SatVariant=Disabled  AWVariant=Disabled  PCopyVariant=Disabled  TRVariant=Disabled  FdbkBlocksVariant=Forward  IdealPFdbkVariant=Disabled  SatFdbkVariant=Disabled  DerivativeFilterVariant=Disabled  NVariant=Disabled  NCopyVariant=Disabled_SignalSpec  FilterICVariant=Disabled  IntegratorICVariant=Disabled  ExternalResetVariant=Disabled  TRSumVariant=Passthrough  SumFdbkVariant=Disabled  SumVariant=Passthrough_P  TsampFilterVariant=InternalTs  TsampNgainVariant=Passthrough  TsampIntegralVariant=Disabled_SignalSpec  ExternalSaturationOutDataTypeStr=Inherit: Same as second input  DerivativeSourceVariant=Disabled  PreIntVariant=InternalPreInt
  Sum : Sum  Inputs=|+-
  Sum1 : Sum  Inputs=|+-
  Sum2 : Sum  Inputs=|+-
  pid : Subsystem
  pid1 : Subsystem
  pid2 : Subsystem
  姿态角误差 : MATLAB Function  TreatAsAtomicUnit=on
  w_phi : Outport
  w_theta : Outport  Port=2
  w_psi : Outport  Port=3
  wires:
  Constant32/1 -> pid/5(kN)
  Sum1/1 -> pid1/1(u)
  Constant31/1 -> pid/4(kD)
  Demux5/1 -> PID Controller3/1
  姿态角误差/1(angle_err) -> Demux5/1  "attE"
  Demux1/1 -> Sum/2
  pid/1(output) -> w_phi/1  "w_phi"
  pid2/1(output) -> w_psi/1  "w_psi"
  Constant35/1 -> pid1/3(kI)
  Constant30/1 -> pid/3(kI)
  Demux1/2 -> Sum1/2
  pid1/1(output) -> w_theta/1  "w_theta"
  pitch_des/1 -> Mux4/2
  Constant27/1 -> pid/2(kP)
  Constant36/1 -> pid1/4(kD)
  Constant49/1 -> pid2/5(kN)
  "[pqr_act"/1 -> Demux1/1
  Gain11/1 -> pid2/7(lo)
  Gain9/1 -> pid/7(lo)
  Demux5/3 -> PID Controller5/1
  Constant33/1 -> pid/6(up), Gain9/1
  Constant24/1 -> PID Controller3/2
  roll_des/1 -> Mux4/1
  Constant41/1 -> pid2/3(kI)
  Constant38/1 -> pid1/5(kN)
  Constant26/1 -> PID Controller5/2
  Demux1/3 -> Sum2/2
  PID Controller3/1 -> Sum/1, Mux/1
  Constant40/1 -> pid2/2(kP)
  yaw_des/1 -> Mux4/3
  Gain10/1 -> pid1/7(lo)
  Constant42/1 -> pid2/4(kD)
  PID Controller4/1 -> Sum1/1, Mux/2
  euler_act/1 -> 姿态角误差/2(angle_meas)
  Constant50/1 -> pid2/6(up), Gain11/1
  PID Controller5/1 -> Sum2/1, Mux/3
  Demux5/2 -> PID Controller4/1
  Sum2/1 -> pid2/1(u)
  Constant25/1 -> PID Controller4/2
  Constant34/1 -> pid1/2(kP)
  Constant39/1 -> Gain10/1, pid1/6(up)
  Constant7/1 -> pid1/8(Reset1), pid/8(Reset1), pid2/8(Reset1)
  Mux4/1 -> 姿态角误差/1(angle_des)  "target_att"
  Sum/1 -> pid/1(u)
  Mux/1 -> ?
